simulink model "IEEE34bus_v2019b_Phasor_DPL"  (R2019b)
settings: Solver=VariableStepAuto  StartTime=0.0  StopTime=100  FixedStep=Ts  RelTol=1e-3
InitFcn:
  | a=1; % Loading Factor
  | Ts=0.1;% For Delay Blocks in Voltage Regulator Controls
  | 
  | % Simulation data for the IEEE 34 Node Test Feeder model
  | mi2km = 1.60934;%  miles to km conversion
  | ft2km = 0.0003048; % feet to km conversion
  | ms2F = 1*1e-6/(2*pi*60);% microsiemens to Farads conversion
  | 
  | %% Configuration 300 - series reactance - ohm/mile
  | R_300 = [1.3368 0.2101 0.2130;0.2101 1.3238 0.2066;0.2130 0.2066 1.3294];
  | X_300 = [1.3343 0.5779 0.5015;0.5779 1.3569 0.4591;0.5015 0.4591 1.3471];
  | % charging susceptance - microsiemens/mile
  | B_300 = [5.3350 -1.5313 -0.9943;-1.5313 5.0979 -0.6212;-0.9943 -0.6212 4.8880];
  | 
  | R_300 = R_300/mi2km;
  | L_300 = (X_300/(2*pi*60))/mi2km;
  | C_300 =(B_300*ms2F)/mi2km;
  | 
  | %% Configuration 301 - series reactance - ohm/mile
  | R_301 = [1.9300 0.2327 0.2359;0.2327 1.9157 0.2288;0.2359 0.2288 1.9219];
  | X_301 = [1.4115 0.6442 0.5691;0.6442 1.4281 0.5238;0.5691 0.5238 1.4209];
  | % charging susceptance - microsiemens/mile
  | B_301 = [5.1207 -1.4364 -0.9402;-1.4364 4.9055 -0.5951;-0.9402 -0.5951 4.7154];
  | 
  | R_301 = R_301/mi2km;
  | L_301 = (X_301/(2*pi*60))/mi2km;
  | C_301 =(B_301*ms2F)/mi2km;
  | 
  | 
  | %% Configuration 302 - series reactance - ohm/mile
  | R_302 = [2.7995 0 0;0 0 0;0 0 0];
  | X_302 = [1.4855 0 0;0 0 0;0 0 0];
  | % charging susceptance - microsiemens/mile
  | B_302 = [4.2251 0 0;0 0 0;0 0 0];
  | 
  | R_302 = R_302/mi2km;
  | L_302 = (X_302/(2*pi*60))/mi2km;
  | C_302 =(B_302*ms2F)/mi2km;
  | 
  | %% Configuration 303 - series reactance - ohm/mile
  | R_303 = [0 0 0;0 2.7995 0;0 0 0];
  | X_303 = [0 0 0;0 1.4855 0;0 0 0];
  | % charging susceptance - microsiemens/mile
  | B_303 = [0 0 0;0 4.2251 0;0 0 0];
  | 
  | R_303 = R_303/mi2km;
  | L_303 = (X_303/(2*pi*60))/mi2km;
  | C_303 =(B_303*ms2F)/mi2km;
  | 
  | %% Configuration 303 - series reactance - ohm/mile
  | R_304 = [0 0 0;0 1.9217 0;0 0 0];
  | X_304 = [0 0 0;0 1.4212 0;0 0 0];
  | % charging susceptance - microsiemens/mile
  | B_304 = [0 0 0;0 4.3637 0;0 0 0];
  | 
  | R_304 = R_304/mi2km;
  | L_304 = (X_304/(2*pi*60))/mi2km;
  | C_304 =(B_304*ms2F)/mi2km;
undefined symbols (not defined in the file or in its folder): find_system, j
libraries: powerlib x239, powerlib_meascontrol x22
(part 2 of 4)

== system IEEE34bus_v2019b_Phasor_DPL/810 ==
  1 : powerlib/Measurements/Three-Phase V-I Measurement  VoltageMeasurement=phase-to-ground  SetLabelV=on  LabelV=V810  Vpu=off  VpuLL=off  CurrentMeasurement=no  SetLabelI=on  LabelI=I634  Ipu=off  Pbase=100e6  Vbase=24900  OutputType=Complex  PhasorSimulation=on  PSBequivalent=0
      settings: SourceProductName=Simscape Electrical
  Ground{1..2,9,12} (4 alike) : powerlib/Elements/Ground  LConnTagsString=a
      settings: SourceProductName=Simscape Electrical
  b : PMIOPort  Side=Left
  B : PMIOPort  Port=2  Side=Right
  connections:
  Ground2/LConn1 -- 1/LConn3
  Ground1/LConn1 -- 1/RConn3
  b/RConn1 -- 1/RConn2
  1/RConn1 -- Ground9/LConn1
  Ground12/LConn1 -- 1/LConn1
  B/RConn1 -- 1/LConn2

== system IEEE34bus_v2019b_Phasor_DPL/818 ==
  1 : powerlib/Measurements/Three-Phase V-I Measurement  VoltageMeasurement=phase-to-ground  SetLabelV=on  LabelV=V818  Vpu=off  VpuLL=off  CurrentMeasurement=no  SetLabelI=on  LabelI=I634  Ipu=off  Pbase=100e6  Vbase=24900  OutputType=Complex  PhasorSimulation=on  PSBequivalent=0
      settings: SourceProductName=Simscape Electrical
  Ground{1..2,9,12} (4 alike) : powerlib/Elements/Ground  LConnTagsString=a
      settings: SourceProductName=Simscape Electrical
  a : PMIOPort  Side=Left
  A : PMIOPort  Port=2  Side=Right
  connections:
  Ground9/LConn1 -- 1/RConn2
  Ground12/LConn1 -- 1/LConn2
  Ground2/LConn1 -- 1/LConn3
  Ground1/LConn1 -- 1/RConn3
  A/RConn1 -- 1/LConn1
  a/RConn1 -- 1/RConn1

== system IEEE34bus_v2019b_Phasor_DPL/820 ==
  1 : powerlib/Measurements/Three-Phase V-I Measurement  VoltageMeasurement=phase-to-ground  SetLabelV=on  LabelV=V820  Vpu=off  VpuLL=off  CurrentMeasurement=no  SetLabelI=on  LabelI=I634  Ipu=off  Pbase=100e6  Vbase=24900  OutputType=Complex  PhasorSimulation=on  PSBequivalent=0
      settings: SourceProductName=Simscape Electrical
  Ground{1..2,9,12} (4 alike) : powerlib/Elements/Ground  LConnTagsString=a
      settings: SourceProductName=Simscape Electrical
  a : PMIOPort  Side=Left
  A : PMIOPort  Port=2  Side=Right
  connections:
  a/RConn1 -- 1/RConn1
  A/RConn1 -- 1/LConn1
  Ground1/LConn1 -- 1/RConn3
  Ground2/LConn1 -- 1/LConn3
  Ground12/LConn1 -- 1/LConn2
  Ground9/LConn1 -- 1/RConn2

== system IEEE34bus_v2019b_Phasor_DPL/822 ==
  1 : powerlib/Measurements/Three-Phase V-I Measurement  VoltageMeasurement=phase-to-ground  SetLabelV=on  LabelV=V822  Vpu=off  VpuLL=off  CurrentMeasurement=no  SetLabelI=on  LabelI=I634  Ipu=off  Pbase=100e6  Vbase=24900  OutputType=Complex  PhasorSimulation=on  PSBequivalent=0
      settings: SourceProductName=Simscape Electrical
  Ground{1..2,9,12} (4 alike) : powerlib/Elements/Ground  LConnTagsString=a
      settings: SourceProductName=Simscape Electrical
  a : PMIOPort  Side=Left
  A : PMIOPort  Port=2  Side=Right
  connections:
  Ground9/LConn1 -- 1/RConn2
  Ground12/LConn1 -- 1/LConn2
  Ground2/LConn1 -- 1/LConn3
  Ground1/LConn1 -- 1/RConn3
  A/RConn1 -- 1/LConn1
  a/RConn1 -- 1/RConn1

== system IEEE34bus_v2019b_Phasor_DPL/826 ==
  1 : powerlib/Measurements/Three-Phase V-I Measurement  VoltageMeasurement=phase-to-ground  SetLabelV=on  LabelV=V826  Vpu=off  VpuLL=off  CurrentMeasurement=no  SetLabelI=on  LabelI=I634  Ipu=off  Pbase=100e6  Vbase=24900  OutputType=Complex  PhasorSimulation=on  PSBequivalent=0
      settings: SourceProductName=Simscape Electrical
  Ground{1..2,9,12} (4 alike) : powerlib/Elements/Ground  LConnTagsString=a
      settings: SourceProductName=Simscape Electrical
  b : PMIOPort  Side=Left
  B : PMIOPort  Port=2  Side=Right
  connections:
  Ground1/LConn1 -- 1/RConn3
  Ground2/LConn1 -- 1/LConn3
  Ground9/LConn1 -- 1/RConn1
  b/RConn1 -- 1/RConn2
  Ground12/LConn1 -- 1/LConn1
  1/LConn2 -- B/RConn1

== system IEEE34bus_v2019b_Phasor_DPL/838 ==
  1 : powerlib/Measurements/Three-Phase V-I Measurement  VoltageMeasurement=phase-to-ground  SetLabelV=on  LabelV=V838  Vpu=off  VpuLL=off  CurrentMeasurement=no  SetLabelI=on  LabelI=I862  Ipu=off  Pbase=100e6  Vbase=24900  OutputType=Complex  PhasorSimulation=on  PSBequivalent=0
      settings: SourceProductName=Simscape Electrical
  Ground{1..2,9,12} (4 alike) : powerlib/Elements/Ground  LConnTagsString=a
      settings: SourceProductName=Simscape Electrical
  b : PMIOPort  Side=Left
  B : PMIOPort  Port=2  Side=Right
  connections:
  1/LConn2 -- B/RConn1
  Ground12/LConn1 -- 1/LConn1
  b/RConn1 -- 1/RConn2
  Ground9/LConn1 -- 1/RConn1
  Ground2/LConn1 -- 1/LConn3
  Ground1/LConn1 -- 1/RConn3

== system IEEE34bus_v2019b_Phasor_DPL/856 ==
  1 : powerlib/Measurements/Three-Phase V-I Measurement  VoltageMeasurement=phase-to-ground  SetLabelV=on  LabelV=V856  Vpu=off  VpuLL=off  CurrentMeasurement=no  SetLabelI=on  LabelI=I634  Ipu=off  Pbase=100e6  Vbase=24900  OutputType=Complex  PhasorSimulation=on  PSBequivalent=0
      settings: SourceProductName=Simscape Electrical
  Ground{1..2,9,12} (4 alike) : powerlib/Elements/Ground  LConnTagsString=a
      settings: SourceProductName=Simscape Electrical
  b : PMIOPort  Side=Left
  B : PMIOPort  Port=2  Side=Right
  connections:
  1/LConn2 -- B/RConn1
  Ground12/LConn1 -- 1/LConn1
  b/RConn1 -- 1/RConn2
  Ground9/LConn1 -- 1/RConn1
  Ground2/LConn1 -- 1/LConn3
  Ground1/LConn1 -- 1/RConn3

== system IEEE34bus_v2019b_Phasor_DPL/864 ==
  1 : powerlib/Measurements/Three-Phase V-I Measurement  VoltageMeasurement=phase-to-ground  SetLabelV=on  LabelV=V864  Vpu=off  VpuLL=off  CurrentMeasurement=no  SetLabelI=on  LabelI=I634  Ipu=off  Pbase=100e6  Vbase=24900  OutputType=Complex  PhasorSimulation=on  PSBequivalent=0
      settings: SourceProductName=Simscape Electrical
  Ground{1..2,9,12} (4 alike) : powerlib/Elements/Ground  LConnTagsString=a
      settings: SourceProductName=Simscape Electrical
  a : PMIOPort  Side=Left
  A : PMIOPort  Port=2  Side=Right
  connections:
  a/RConn1 -- 1/RConn1
  A/RConn1 -- 1/LConn1
  Ground1/LConn1 -- 1/RConn3
  Ground2/LConn1 -- 1/LConn3
  Ground12/LConn1 -- 1/LConn2
  Ground9/LConn1 -- 1/RConn2

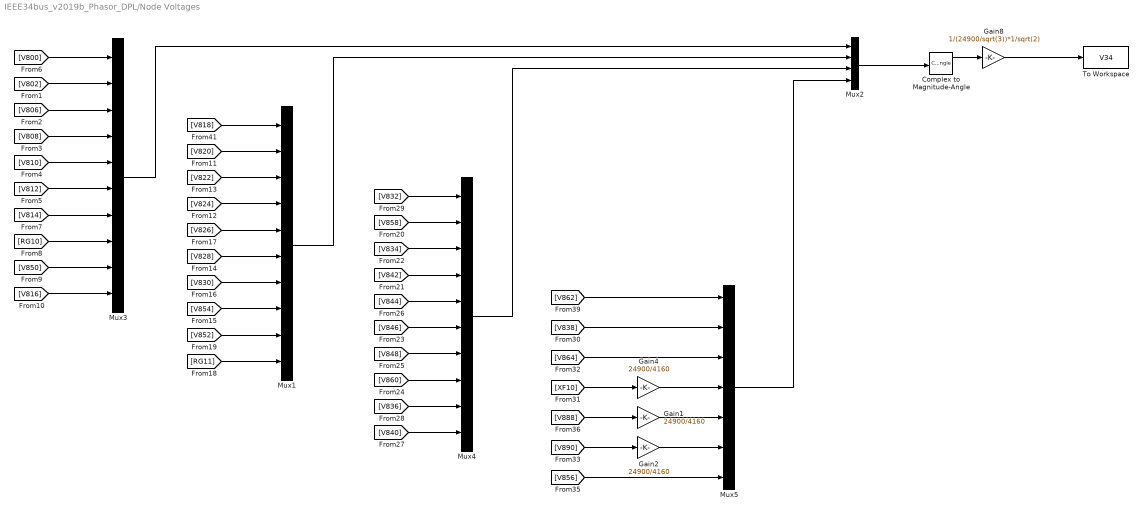
== system IEEE34bus_v2019b_Phasor_DPL/Node Voltages ==
  Complex to Magnitude-Angle : ComplexToMagnitudeAngle
  Gain1 : Gain  Gain=24900/4160
  Gain2 : Gain  Gain=24900/4160
  Gain4 : Gain  Gain=24900/4160
  Gain8 : Gain  Gain=1/(24900/sqrt(3))*1/sqrt(2)
  Mux1 : Mux  Inputs=10
  Mux2 : Mux
  Mux3 : Mux  Inputs=10
  Mux4 : Mux  Inputs=10
  Mux5 : Mux  Inputs=7
  To Workspace : ToWorkspace  VariableName=V34  SampleTime=0.1
  wires:
  [V800] -> Mux3/1
  [V802] -> Mux3/2
  [V806] -> Mux3/3
  [V808] -> Mux3/4
  [V810] -> Mux3/5
  [V812] -> Mux3/6
  [V814] -> Mux3/7
  [RG10] -> Mux3/8
  [V850] -> Mux3/9
  [V816] -> Mux3/10
  [V818] -> Mux1/1
  [V820] -> Mux1/2
  [V822] -> Mux1/3
  [V824] -> Mux1/4
  [V826] -> Mux1/5
  [V828] -> Mux1/6
  [V830] -> Mux1/7
  [V854] -> Mux1/8
  [V852] -> Mux1/9
  [RG11] -> Mux1/10
  [V832] -> Mux4/1
  [V858] -> Mux4/2
  [V834] -> Mux4/3
  [V842] -> Mux4/4
  [V844] -> Mux4/5
  [V846] -> Mux4/6
  [V848] -> Mux4/7
  [V860] -> Mux4/8
  [V836] -> Mux4/9
  [V840] -> Mux4/10
  [V862] -> Mux5/1
  [V838] -> Mux5/2
  [V864] -> Mux5/3
  [XF10] -> Gain4/1
  [V888] -> Gain1/1
  [V890] -> Gain2/1
  [V856] -> Mux5/7
  Mux3/1 -> Mux2/1
  Mux1/1 -> Mux2/2
  Mux4/1 -> Mux2/3
  Mux5/1 -> Mux2/4
  Gain4/1 -> Mux5/4
  Gain1/1 -> Mux5/5
  Gain2/1 -> Mux5/6
  Gain8/1 -> To Workspace/1
  Complex to Magnitude-Angle/1 -> Gain8/1
  Mux2/1 -> Complex to Magnitude-Angle/1

== system IEEE34bus_v2019b_Phasor_DPL/Regulator 1 ==
  Mux : Mux  Inputs=3
  Single Phase SVR_A : Subsystem  LoadFcn=find_system(gcs,'FollowLinks', 'on', 'LookUnderMasks', 'all');  mask(Single-Phase OLTC){pNom=5e6/3, fNom=60, vNom=24.9e3/sqrt(3), ctRatio=100, ptRatio=120, DeltaU=0.00625, TapMinMax=[-16 16], InitialTap=12, TapSelectionTime=8, RegulatorOn=on, Regulator=[122/120  2/120  2], Comp=[2.7 1.6]}
      mask prompts: pNom "Nominal Power (VA)"; fNom "Nominal Frequency (Hz)"; vNom "Nominal Voltage (Vrms)"; ctRatio "Primary CT Rating (A)"; ptRatio "PT Ratio"; DeltaU "Voltage Step Per Tap (pu)"; TapMinMax "Minimum and Maximum Tap Positions"; InitialTap "Initial Tap Position"; TapSelectionTime "Tap Selection Time (s)"; RegulatorOn "Voltage Regulator"; Regulator "Voltage Regulator [ Vref(pu) DeadBand(pu)  Delay(s)]"; Comp "Compensator Settings [R (V) X(V)]"
      mask help:
      | Models a single-phase On Load Tap Changer (OLTC). The single-phase primary of multi-tap winding is modeled with a Variable-Ratio Transformer block.
      |
      | The transformer voltage ratio U2/U1 (in pu) is given by:
      |                 U2/U1= 1/ (1+TapPosition*DeltaU)
      | Tap position 0 corresponds to nominal voltage ratio.
      |
      | When Voltage regulator is 'on',  voltage regulator asks for a tap change if:
      |                  abs(Vm-Vref)>DeadBand/2  during a time  t > Delay.
      |
      | where 'Vm' is voltage measured at regulating point and Vref is reference voltage.
      | With line drop compensation, Vm=Vsec-Isec(R+jX)
      mask init:
      | RegulatorVref=Regulator(1);
      | RegulatorDeadBand=Regulator(2);
      | RegulatorDelay=Regulator(3);
      | Rc=Comp(1);
      | Xc=Comp(2);
      mask TypeOptions RegulatorOn: off | on
      mask Callback RegulatorOn:
      | tempMaskVis=get_param(gcb,'MaskVisibilities');
      | if strcmp(get_param(gcb,'RegulatorOn'),'on')
      | 	tempMaskVis{11}='on';
      | 	set_param(gcb,'MaskVisibilities',tempMaskVis);
      | else
      | 	tempMaskVis{11}='off';
      | 	set_param(gcb,'MaskVisibilities',tempMaskVis);
      | end
      | if strcmp(get_param(gcb,'RegulatorOn'),'on')
      | 	tempMaskVis{12}='on';
      | 	set_param(gcb,'MaskVisibilities',tempMaskVis);
      | else
      | 	tempMaskVis{12}='off';
      | 	set_param(gcb,'MaskVisibilities',tempMaskVis);
      | end
      mask DialogControl Container8 Prompt: Setup
      mask DialogControl Container13 Prompt: Regulator Parameters
  Single Phase SVR_B : Subsystem  LoadFcn=find_system(gcs,'FollowLinks', 'on', 'LookUnderMasks', 'all');  mask(Single-Phase OLTC){pNom=5e6/3, fNom=60, vNom=24.9e3/sqrt(3), ctRatio=100, ptRatio=120, DeltaU=0.00625, TapMinMax=[-16 16], InitialTap=5, TapSelectionTime=8, RegulatorOn=on, Regulator=[122/120  2/120  2], Comp=[2.7 1.6]}
      mask prompts: pNom "Nominal Power (VA)"; fNom "Nominal Frequency (Hz)"; vNom "Nominal Voltage (Vrms)"; ctRatio "Primary CT Rating (A)"; ptRatio "PT Ratio"; DeltaU "Voltage Step Per Tap (pu)"; TapMinMax "Minimum and Maximum Tap Positions"; InitialTap "Initial Tap Position"; TapSelectionTime "Tap Selection Time (s)"; RegulatorOn "Voltage Regulator"; Regulator "Voltage Regulator [ Vref(pu) DeadBand(pu)  Delay(s)]"; Comp "Compensator Settings [R (V) X(V)]"
      mask help:
      | Models a single-phase On Load Tap Changer (OLTC). The single-phase primary of multi-tap winding is modeled with a Variable-Ratio Transformer block.
      |
      | The transformer voltage ratio U2/U1 (in pu) is given by:
      |                 U2/U1= 1/ (1+TapPosition*DeltaU)
      | Tap position 0 corresponds to nominal voltage ratio.
      |
      | When Voltage regulator is 'on',  voltage regulator asks for a tap change if:
      |                  abs(Vm-Vref)>DeadBand/2  during a time  t > Delay.
      |
      | where 'Vm' is voltage measured at regulating point and Vref is reference voltage.
      | With line drop compensation, Vm=Vsec-Isec(R+jX)
      mask init:
      | RegulatorVref=Regulator(1);
      | RegulatorDeadBand=Regulator(2);
      | RegulatorDelay=Regulator(3);
      | Rc=Comp(1);
      | Xc=Comp(2);
      mask TypeOptions RegulatorOn: off | on
      mask Callback RegulatorOn:
      | tempMaskVis=get_param(gcb,'MaskVisibilities');
      | if strcmp(get_param(gcb,'RegulatorOn'),'on')
      | 	tempMaskVis{11}='on';
      | 	set_param(gcb,'MaskVisibilities',tempMaskVis);
      | else
      | 	tempMaskVis{11}='off';
      | 	set_param(gcb,'MaskVisibilities',tempMaskVis);
      | end
      | if strcmp(get_param(gcb,'RegulatorOn'),'on')
      | 	tempMaskVis{12}='on';
      | 	set_param(gcb,'MaskVisibilities',tempMaskVis);
      | else
      | 	tempMaskVis{12}='off';
      | 	set_param(gcb,'MaskVisibilities',tempMaskVis);
      | end
      mask DialogControl Container8 Prompt: Setup
      mask DialogControl Container13 Prompt: Regulator Parameters
  Single Phase SVR_C : Subsystem  LoadFcn=find_system(gcs,'FollowLinks', 'on', 'LookUnderMasks', 'all');  mask(Single-Phase OLTC){pNom=5e6/3, fNom=60, vNom=24.9e3/sqrt(3), ctRatio=100, ptRatio=120, DeltaU=0.00625, TapMinMax=[-16 16], InitialTap=5, TapSelectionTime=8, RegulatorOn=on, Regulator=[122/120  2/120  2], Comp=[2.7 1.6]}
      mask prompts: pNom "Nominal Power (VA)"; fNom "Nominal Frequency (Hz)"; vNom "Nominal Voltage (Vrms)"; ctRatio "Primary CT Rating (A)"; ptRatio "PT Ratio"; DeltaU "Voltage Step Per Tap (pu)"; TapMinMax "Minimum and Maximum Tap Positions"; InitialTap "Initial Tap Position"; TapSelectionTime "Tap Selection Time (s)"; RegulatorOn "Voltage Regulator"; Regulator "Voltage Regulator [ Vref(pu) DeadBand(pu)  Delay(s)]"; Comp "Compensator Settings [R (V) X(V)]"
      mask help:
      | Models a single-phase On Load Tap Changer (OLTC). The single-phase primary of multi-tap winding is modeled with a Variable-Ratio Transformer block.
      |
      | The transformer voltage ratio U2/U1 (in pu) is given by:
      |                 U2/U1= 1/ (1+TapPosition*DeltaU)
      | Tap position 0 corresponds to nominal voltage ratio.
      |
      | When Voltage regulator is 'on',  voltage regulator asks for a tap change if:
      |                  abs(Vm-Vref)>DeadBand/2  during a time  t > Delay.
      |
      | where 'Vm' is voltage measured at regulating point and Vref is reference voltage.
      | With line drop compensation, Vm=Vsec-Isec(R+jX)
      mask init:
      | RegulatorVref=Regulator(1);
      | RegulatorDeadBand=Regulator(2);
      | RegulatorDelay=Regulator(3);
      | Rc=Comp(1);
      | Xc=Comp(2);
      mask TypeOptions RegulatorOn: off | on
      mask Callback RegulatorOn:
      | tempMaskVis=get_param(gcb,'MaskVisibilities');
      | if strcmp(get_param(gcb,'RegulatorOn'),'on')
      | 	tempMaskVis{11}='on';
      | 	set_param(gcb,'MaskVisibilities',tempMaskVis);
      | else
      | 	tempMaskVis{11}='off';
      | 	set_param(gcb,'MaskVisibilities',tempMaskVis);
      | end
      | if strcmp(get_param(gcb,'RegulatorOn'),'on')
      | 	tempMaskVis{12}='on';
      | 	set_param(gcb,'MaskVisibilities',tempMaskVis);
      | else
      | 	tempMaskVis{12}='off';
      | 	set_param(gcb,'MaskVisibilities',tempMaskVis);
      | end
      mask DialogControl Container8 Prompt: Setup
      mask DialogControl Container13 Prompt: Regulator Parameters
  A : PMIOPort  Side=Left
  a : PMIOPort  Port=2  Side=Right
  B : PMIOPort  Port=3  Side=Left
  b : PMIOPort  Port=4  Side=Right
  C : PMIOPort  Port=5  Side=Left
  c : PMIOPort  Port=6  Side=Right
  Tap : Outport
  wires:
  Mux/1 -> Tap/1
  Single Phase SVR_C/1(Tap) -> Mux/3
  Single Phase SVR_B/1(Tap) -> Mux/2
  Single Phase SVR_A/1(Tap) -> Mux/1
  connections:
  Single Phase SVR_C/RConn1 -- c/RConn1
  Single Phase SVR_C/LConn1 -- C/RConn1
  Single Phase SVR_B/RConn1 -- b/RConn1
  Single Phase SVR_B/LConn1 -- B/RConn1
  Single Phase SVR_A/LConn1 -- A/RConn1
  Single Phase SVR_A/RConn1 -- a/RConn1

== system IEEE34bus_v2019b_Phasor_DPL/Regulator 2 ==
  Mux : Mux  Inputs=3
  Single Phase SVR_A : Subsystem  LoadFcn=find_system(gcs,'FollowLinks', 'on', 'LookUnderMasks', 'all');  mask(Single-Phase OLTC){pNom=5e6/3, fNom=60, vNom=24.9e3/sqrt(3), ctRatio=100, ptRatio=120, DeltaU=0.00625, TapMinMax=[-16 16], InitialTap=13, TapSelectionTime=13, RegulatorOn=on, Regulator=[124/120  2/120  2], Comp=[2.5 1.5]}
      mask prompts: pNom "Nominal Power (VA)"; fNom "Nominal Frequency (Hz)"; vNom "Nominal Voltage (Vrms)"; ctRatio "Primary CT Rating (A)"; ptRatio "PT Ratio"; DeltaU "Voltage Step Per Tap (pu)"; TapMinMax "Minimum and Maximum Tap Positions"; InitialTap "Initial Tap Position"; TapSelectionTime "Tap Selection Time (s)"; RegulatorOn "Voltage Regulator"; Regulator "Voltage Regulator [ Vref(pu) DeadBand(pu)  Delay(s)]"; Comp "Compensator Settings [R (V) X(V)]"
      mask help:
      | Models a single-phase On Load Tap Changer (OLTC). The single-phase primary of multi-tap winding is modeled with a Variable-Ratio Transformer block.
      |
      | The transformer voltage ratio U2/U1 (in pu) is given by:
      |                 U2/U1= 1/ (1+TapPosition*DeltaU)
      | Tap position 0 corresponds to nominal voltage ratio.
      |
      | When Voltage regulator is 'on',  voltage regulator asks for a tap change if:
      |                  abs(Vm-Vref)>DeadBand/2  during a time  t > Delay.
      |
      | where 'Vm' is voltage measured at regulating point and Vref is reference voltage.
      | With line drop compensation, Vm=Vsec-Isec(R+jX)
      mask init:
      | RegulatorVref=Regulator(1);
      | RegulatorDeadBand=Regulator(2);
      | RegulatorDelay=Regulator(3);
      | Rc=Comp(1);
      | Xc=Comp(2);
      mask TypeOptions RegulatorOn: off | on
      mask Callback RegulatorOn:
      | tempMaskVis=get_param(gcb,'MaskVisibilities');
      | if strcmp(get_param(gcb,'RegulatorOn'),'on')
      | 	tempMaskVis{11}='on';
      | 	set_param(gcb,'MaskVisibilities',tempMaskVis);
      | else
      | 	tempMaskVis{11}='off';
      | 	set_param(gcb,'MaskVisibilities',tempMaskVis);
      | end
      | if strcmp(get_param(gcb,'RegulatorOn'),'on')
      | 	tempMaskVis{12}='on';
      | 	set_param(gcb,'MaskVisibilities',tempMaskVis);
      | else
      | 	tempMaskVis{12}='off';
      | 	set_param(gcb,'MaskVisibilities',tempMaskVis);
      | end
      mask DialogControl Container8 Prompt: Setup
      mask DialogControl Container13 Prompt: Regulator Parameters
  Single Phase SVR_B : Subsystem  LoadFcn=find_system(gcs,'FollowLinks', 'on', 'LookUnderMasks', 'all');  mask(Single-Phase OLTC){pNom=5e6/3, fNom=60, vNom=24.9e3/sqrt(3), ctRatio=100, ptRatio=120, DeltaU=0.00625, TapMinMax=[-16 16], InitialTap=11, TapSelectionTime=13, RegulatorOn=on, Regulator=[124/120  2/120  2], Comp=[2.5 1.5]}
      mask prompts: pNom "Nominal Power (VA)"; fNom "Nominal Frequency (Hz)"; vNom "Nominal Voltage (Vrms)"; ctRatio "Primary CT Rating (A)"; ptRatio "PT Ratio"; DeltaU "Voltage Step Per Tap (pu)"; TapMinMax "Minimum and Maximum Tap Positions"; InitialTap "Initial Tap Position"; TapSelectionTime "Tap Selection Time (s)"; RegulatorOn "Voltage Regulator"; Regulator "Voltage Regulator [ Vref(pu) DeadBand(pu)  Delay(s)]"; Comp "Compensator Settings [R (V) X(V)]"
      mask help:
      | Models a single-phase On Load Tap Changer (OLTC). The single-phase primary of multi-tap winding is modeled with a Variable-Ratio Transformer block.
      |
      | The transformer voltage ratio U2/U1 (in pu) is given by:
      |                 U2/U1= 1/ (1+TapPosition*DeltaU)
      | Tap position 0 corresponds to nominal voltage ratio.
      |
      | When Voltage regulator is 'on',  voltage regulator asks for a tap change if:
      |                  abs(Vm-Vref)>DeadBand/2  during a time  t > Delay.
      |
      | where 'Vm' is voltage measured at regulating point and Vref is reference voltage.
      | With line drop compensation, Vm=Vsec-Isec(R+jX)
      mask init:
      | RegulatorVref=Regulator(1);
      | RegulatorDeadBand=Regulator(2);
      | RegulatorDelay=Regulator(3);
      | Rc=Comp(1);
      | Xc=Comp(2);
      mask TypeOptions RegulatorOn: off | on
      mask Callback RegulatorOn:
      | tempMaskVis=get_param(gcb,'MaskVisibilities');
      | if strcmp(get_param(gcb,'RegulatorOn'),'on')
      | 	tempMaskVis{11}='on';
      | 	set_param(gcb,'MaskVisibilities',tempMaskVis);
      | else
      | 	tempMaskVis{11}='off';
      | 	set_param(gcb,'MaskVisibilities',tempMaskVis);
      | end
      | if strcmp(get_param(gcb,'RegulatorOn'),'on')
      | 	tempMaskVis{12}='on';
      | 	set_param(gcb,'MaskVisibilities',tempMaskVis);
      | else
      | 	tempMaskVis{12}='off';
      | 	set_param(gcb,'MaskVisibilities',tempMaskVis);
      | end
      mask DialogControl Container8 Prompt: Setup
      mask DialogControl Container13 Prompt: Regulator Parameters
  Single Phase SVR_C : Subsystem  LoadFcn=find_system(gcs,'FollowLinks', 'on', 'LookUnderMasks', 'all');  mask(Single-Phase OLTC){pNom=5e6/3, fNom=60, vNom=24.9e3/sqrt(3), ctRatio=100, ptRatio=120, DeltaU=0.00625, TapMinMax=[-16 16], InitialTap=12, TapSelectionTime=13, RegulatorOn=on, Regulator=[124/120  2/120  2], Comp=[2.5 1.5]}
      mask prompts: pNom "Nominal Power (VA)"; fNom "Nominal Frequency (Hz)"; vNom "Nominal Voltage (Vrms)"; ctRatio "Primary CT Rating (A)"; ptRatio "PT Ratio"; DeltaU "Voltage Step Per Tap (pu)"; TapMinMax "Minimum and Maximum Tap Positions"; InitialTap "Initial Tap Position"; TapSelectionTime "Tap Selection Time (s)"; RegulatorOn "Voltage Regulator"; Regulator "Voltage Regulator [ Vref(pu) DeadBand(pu)  Delay(s)]"; Comp "Compensator Settings [R (V) X(V)]"
      mask help:
      | Models a single-phase On Load Tap Changer (OLTC). The single-phase primary of multi-tap winding is modeled with a Variable-Ratio Transformer block.
      |
      | The transformer voltage ratio U2/U1 (in pu) is given by:
      |                 U2/U1= 1/ (1+TapPosition*DeltaU)
      | Tap position 0 corresponds to nominal voltage ratio.
      |
      | When Voltage regulator is 'on',  voltage regulator asks for a tap change if:
      |                  abs(Vm-Vref)>DeadBand/2  during a time  t > Delay.
      |
      | where 'Vm' is voltage measured at regulating point and Vref is reference voltage.
      | With line drop compensation, Vm=Vsec-Isec(R+jX)
      mask init:
      | RegulatorVref=Regulator(1);
      | RegulatorDeadBand=Regulator(2);
      | RegulatorDelay=Regulator(3);
      | Rc=Comp(1);
      | Xc=Comp(2);
      mask TypeOptions RegulatorOn: off | on
      mask Callback RegulatorOn:
      | tempMaskVis=get_param(gcb,'MaskVisibilities');
      | if strcmp(get_param(gcb,'RegulatorOn'),'on')
      | 	tempMaskVis{11}='on';
      | 	set_param(gcb,'MaskVisibilities',tempMaskVis);
      | else
      | 	tempMaskVis{11}='off';
      | 	set_param(gcb,'MaskVisibilities',tempMaskVis);
      | end
      | if strcmp(get_param(gcb,'RegulatorOn'),'on')
      | 	tempMaskVis{12}='on';
      | 	set_param(gcb,'MaskVisibilities',tempMaskVis);
      | else
      | 	tempMaskVis{12}='off';
      | 	set_param(gcb,'MaskVisibilities',tempMaskVis);
      | end
      mask DialogControl Container8 Prompt: Setup
      mask DialogControl Container13 Prompt: Regulator Parameters
  A : PMIOPort  Side=Left
  a : PMIOPort  Port=2  Side=Right
  B : PMIOPort  Port=3  Side=Left
  b : PMIOPort  Port=4  Side=Right
  C : PMIOPort  Port=5  Side=Left
  c : PMIOPort  Port=6  Side=Right
  Tap : Outport
  wires:
  Mux/1 -> Tap/1
  Single Phase SVR_C/1(Tap) -> Mux/3
  Single Phase SVR_B/1(Tap) -> Mux/2
  Single Phase SVR_A/1(Tap) -> Mux/1
  connections:
  Single Phase SVR_C/RConn1 -- c/RConn1
  Single Phase SVR_C/LConn1 -- C/RConn1
  Single Phase SVR_B/RConn1 -- b/RConn1
  Single Phase SVR_B/LConn1 -- B/RConn1
  Single Phase SVR_A/LConn1 -- A/RConn1
  Single Phase SVR_A/RConn1 -- a/RConn1

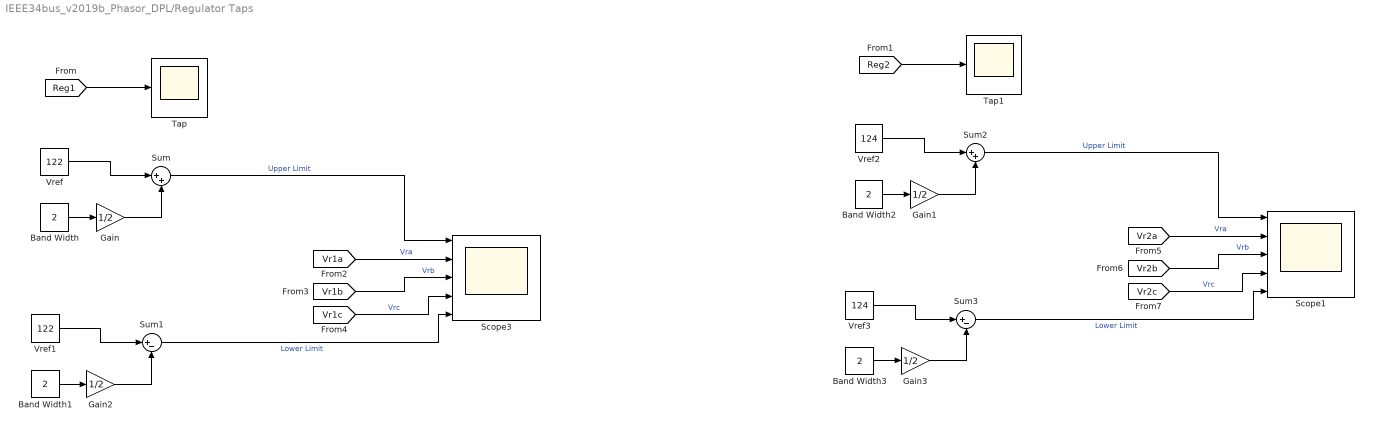
== system IEEE34bus_v2019b_Phasor_DPL/Regulator Taps ==
  Band Width{,1..3} (4 alike) : Constant  Value=2
  Gain{,1..3} (4 alike) : Gain  Gain=1/2
  Scope1 : Scope  NumInputPorts=5
  Scope3 : Scope  NumInputPorts=5
  Sum : Sum  Inputs=|++
  Sum1 : Sum  Inputs=|+-
  Sum2 : Sum  Inputs=|++
  Sum3 : Sum  Inputs=|+-
  Tap : Scope
  Tap1 : Scope
  Vref : Constant  Value=122
  Vref1 : Constant  Value=122
  Vref2 : Constant  Value=124
  Vref3 : Constant  Value=124
  wires:
  Vref/1 -> Sum/1
  Gain2/1 -> Sum1/2
  Band Width/1 -> Gain/1
  Gain/1 -> Sum/2
  [Reg1] -> Tap/1
  [Vr1c] -> Scope3/4  "Vrc"
  Band Width1/1 -> Gain2/1
  Sum/1 -> Scope3/1  "Upper Limit"
  Vref1/1 -> Sum1/1
  Sum1/1 -> Scope3/5  "Lower Limit"
  [Vr1b] -> Scope3/3  "Vrb"
  [Vr1a] -> Scope3/2  "Vra"
  [Vr2a] -> Scope1/2  "Vra"
  [Vr2b] -> Scope1/3  "Vrb"
  Sum3/1 -> Scope1/5  "Lower Limit"
  Vref3/1 -> Sum3/1
  Sum2/1 -> Scope1/1  "Upper Limit"
  Band Width3/1 -> Gain3/1
  [Vr2c] -> Scope1/4  "Vrc"
  [Reg2] -> Tap1/1
  Gain1/1 -> Sum2/2
  Band Width2/1 -> Gain1/1
  Gain3/1 -> Sum3/2
  Vref2/1 -> Sum2/1

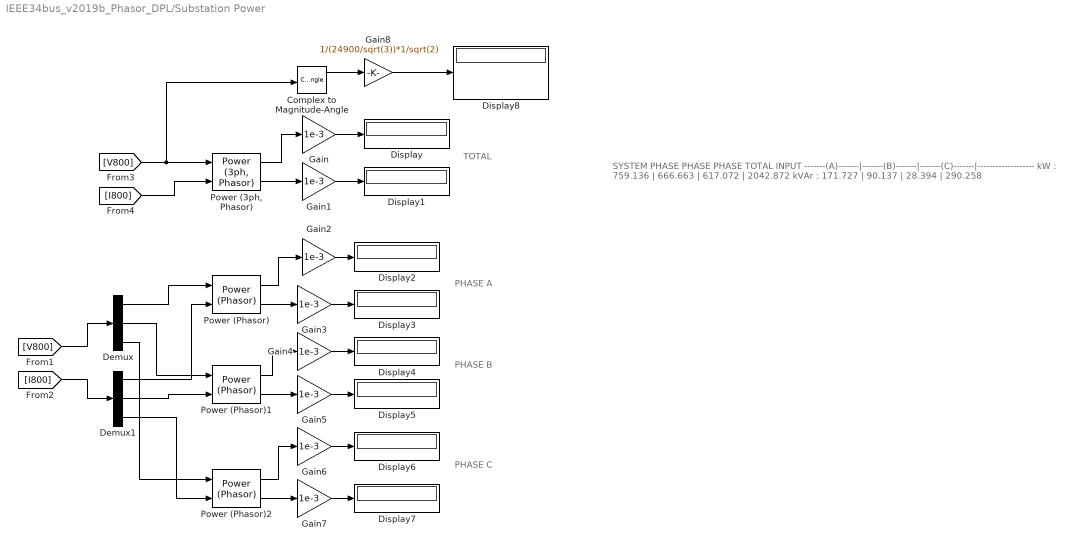
== system IEEE34bus_v2019b_Phasor_DPL/Substation Power ==
  note: SYSTEM PHASE PHASE PHASE TOTAL
      | INPUT -------(A)-------|-------(B)-------|-------(C)-------|-------------------
      | kW : 759.136 | 666.663 | 617.072 | 2042.872
      | kVAr : 171.727 | 90.137 | 28.394 | 290.258
  note: PHASE C
  note: PHASE A
  note: PHASE B
  note: TOTAL
  Complex to Magnitude-Angle : ComplexToMagnitudeAngle
  Demux : Demux  Outputs=3
  Demux1 : Demux  Outputs=3
  Display{,1..8} (9 alike) : Display
  Gain{,1..7} (8 alike) : Gain  Gain=1e-3
  Gain8 : Gain  Gain=1/(24900/sqrt(3))*1/sqrt(2)
  "Power (3ph, Phasor)" : powerlib_meascontrol/Measurements/Power (3ph, Phasor)
      settings: SourceProductName=Simscape Electrical  SourceProductBaseCode=PS
  Power (Phasor) : powerlib_meascontrol/Measurements/Power (Phasor)
      settings: SourceProductName=Simscape Electrical  SourceProductBaseCode=PS
  Power (Phasor)1 : powerlib_meascontrol/Measurements/Power (Phasor)
      settings: SourceProductName=Simscape Electrical  SourceProductBaseCode=PS
  Power (Phasor)2 : powerlib_meascontrol/Measurements/Power (Phasor)
      settings: SourceProductName=Simscape Electrical  SourceProductBaseCode=PS
  wires:
  [I800] -> "Power (3ph, Phasor)"/2
  "Power (3ph, Phasor)"/1 -> Gain/1
  "Power (3ph, Phasor)"/2 -> Gain1/1
  [V800] -> Demux/1
  [I800] -> Demux1/1
  Demux/1 -> Power (Phasor)/1
  Demux1/1 -> Power (Phasor)/2
  Demux/2 -> Power (Phasor)1/1
  Demux1/2 -> Power (Phasor)1/2
  Demux/3 -> Power (Phasor)2/1
  Demux1/3 -> Power (Phasor)2/2
  Power (Phasor)/1 -> Gain2/1
  Power (Phasor)/2 -> Gain3/1
  Power (Phasor)1/1 -> Gain4/1
  Power (Phasor)1/2 -> Gain5/1
  Power (Phasor)2/1 -> Gain6/1
  Power (Phasor)2/2 -> Gain7/1
  Gain/1 -> Display/1
  Gain1/1 -> Display1/1
  Gain2/1 -> Display2/1
  Gain3/1 -> Display3/1
  Gain4/1 -> Display4/1
  Gain5/1 -> Display5/1
  Gain6/1 -> Display6/1
  Gain7/1 -> Display7/1
  Complex to Magnitude-Angle/1 -> Gain8/1
  [V800] -> Complex to Magnitude-Angle/1, "Power (3ph, Phasor)"/1
  Gain8/1 -> Display8/1

== system IEEE34bus_v2019b_Phasor_DPL/Regulator 1/Single Phase SVR_A ==
  Line Drop Compensator : Subsystem
  Transformer with Taps : Subsystem
  Voltage Regulator Control : Subsystem
  S : PMIOPort  Tag=PMCPort  Side=Left
  L : PMIOPort  Tag=PMCPort  Port=2  Side=Right
  Tap : Outport  VectorParamsAs1DForOutWhenUnconnected=off
  tag scope: Vr1a=global
  wires:
  Line Drop Compensator/1(Vm) -> [Vr1a], Voltage Regulator Control/1(Vm)
  Voltage Regulator Control/1(Tap) -> Transformer with Taps/1(tap), Tap/1
  Transformer with Taps/1(Isec) -> Line Drop Compensator/1(Isec)
  Transformer with Taps/2(Vsec) -> Line Drop Compensator/2(Vsec)
  connections:
  Transformer with Taps/RConn1 -- L/RConn1
  Transformer with Taps/LConn1 -- S/RConn1

== system IEEE34bus_v2019b_Phasor_DPL/Regulator 1/Single Phase SVR_B ==
  Line Drop Compensator : Subsystem
  Transformer with Taps : Subsystem
  Voltage Regulator Control : Subsystem
  S : PMIOPort  Tag=PMCPort  Side=Left
  L : PMIOPort  Tag=PMCPort  Port=2  Side=Right
  Tap : Outport  VectorParamsAs1DForOutWhenUnconnected=off
  tag scope: Vr1b=global
  wires:
  Transformer with Taps/2(Vsec) -> Line Drop Compensator/2(Vsec)
  Transformer with Taps/1(Isec) -> Line Drop Compensator/1(Isec)
  Voltage Regulator Control/1(Tap) -> Transformer with Taps/1(tap), Tap/1
  Line Drop Compensator/1(Vm) -> [Vr1b], Voltage Regulator Control/1(Vm)
  connections:
  Transformer with Taps/LConn1 -- S/RConn1
  Transformer with Taps/RConn1 -- L/RConn1

== system IEEE34bus_v2019b_Phasor_DPL/Regulator 1/Single Phase SVR_C ==
  Line Drop Compensator : Subsystem
  Transformer with Taps : Subsystem
  Voltage Regulator Control : Subsystem
  S : PMIOPort  Tag=PMCPort  Side=Left
  L : PMIOPort  Tag=PMCPort  Port=2  Side=Right
  Tap : Outport  VectorParamsAs1DForOutWhenUnconnected=off
  tag scope: Vr1c=global
  wires:
  Line Drop Compensator/1(Vm) -> [Vr1c], Voltage Regulator Control/1(Vm)
  Voltage Regulator Control/1(Tap) -> Transformer with Taps/1(tap), Tap/1
  Transformer with Taps/1(Isec) -> Line Drop Compensator/1(Isec)
  Transformer with Taps/2(Vsec) -> Line Drop Compensator/2(Vsec)
  connections:
  Transformer with Taps/RConn1 -- L/RConn1
  Transformer with Taps/LConn1 -- S/RConn1

== system IEEE34bus_v2019b_Phasor_DPL/Regulator 2/Single Phase SVR_A ==
  Line Drop Compensator : Subsystem
  Transformer with Taps : Subsystem
  Voltage Regulator Control : Subsystem
  S : PMIOPort  Tag=PMCPort  Side=Left
  L : PMIOPort  Tag=PMCPort  Port=2  Side=Right
  Tap : Outport  VectorParamsAs1DForOutWhenUnconnected=off
  tag scope: Vr2a=global
  wires:
  Line Drop Compensator/1(Vm) -> [Vr2a], Voltage Regulator Control/1(Vm)
  Voltage Regulator Control/1(Tap) -> Transformer with Taps/1(tap), Tap/1
  Transformer with Taps/1(Isec) -> Line Drop Compensator/1(Isec)
  Transformer with Taps/2(Vsec) -> Line Drop Compensator/2(Vsec)
  connections:
  Transformer with Taps/RConn1 -- L/RConn1
  Transformer with Taps/LConn1 -- S/RConn1

== system IEEE34bus_v2019b_Phasor_DPL/Regulator 2/Single Phase SVR_B ==
  Line Drop Compensator : Subsystem
  Transformer with Taps : Subsystem
  Voltage Regulator Control : Subsystem
  S : PMIOPort  Tag=PMCPort  Side=Left
  L : PMIOPort  Tag=PMCPort  Port=2  Side=Right
  Tap : Outport  VectorParamsAs1DForOutWhenUnconnected=off
  tag scope: Vr2b=global
  wires:
  Transformer with Taps/2(Vsec) -> Line Drop Compensator/2(Vsec)
  Transformer with Taps/1(Isec) -> Line Drop Compensator/1(Isec)
  Voltage Regulator Control/1(Tap) -> Transformer with Taps/1(tap), Tap/1
  Line Drop Compensator/1(Vm) -> [Vr2b], Voltage Regulator Control/1(Vm)
  connections:
  Transformer with Taps/LConn1 -- S/RConn1
  Transformer with Taps/RConn1 -- L/RConn1

== system IEEE34bus_v2019b_Phasor_DPL/Regulator 2/Single Phase SVR_C ==
  Line Drop Compensator : Subsystem
  Transformer with Taps : Subsystem
  Voltage Regulator Control : Subsystem
  S : PMIOPort  Tag=PMCPort  Side=Left
  L : PMIOPort  Tag=PMCPort  Port=2  Side=Right
  Tap : Outport  VectorParamsAs1DForOutWhenUnconnected=off
  tag scope: Vr2c=global
  wires:
  Line Drop Compensator/1(Vm) -> [Vr2c], Voltage Regulator Control/1(Vm)
  Voltage Regulator Control/1(Tap) -> Transformer with Taps/1(tap), Tap/1
  Transformer with Taps/1(Isec) -> Line Drop Compensator/1(Isec)
  Transformer with Taps/2(Vsec) -> Line Drop Compensator/2(Vsec)
  connections:
  Transformer with Taps/RConn1 -- L/RConn1
  Transformer with Taps/LConn1 -- S/RConn1

== system IEEE34bus_v2019b_Phasor_DPL/Regulator 1/Single Phase SVR_A/Line Drop Compensator ==
  note: Vm=Vsec-Isec(Rc+jXc)
  Isec : Inport
  Vsec : Inport  Port=2
  Abs1 : Abs
  Gain4 : Gain  Gain=1/sqrt(2)
  Gain5 : Gain  Gain=Rc+j*Xc
  Gain6 : Gain  Gain=1/sqrt(2)
  Sum1 : Sum  Inputs=|+-
  Vm : Outport
  wires:
  Abs1/1 -> Vm/1
  Sum1/1 -> Abs1/1
  Isec/1 -> Gain4/1
  Vsec/1 -> Gain6/1
  Gain4/1 -> Gain5/1
  Gain6/1 -> Sum1/1
  Gain5/1 -> Sum1/2

== system IEEE34bus_v2019b_Phasor_DPL/Regulator 1/Single Phase SVR_A/Transformer with Taps ==
  note: Isec on CT Ratio base
  note: Vsec on Pt Ratio base
  tap : Inport
  "    " : Gain  Gain=(1/ptRatio)
  " 1" : Gain  Gain=(1/ctRatio)
  CT : powerlib/Measurements/Current Measurement  PhasorSimulation=on  OutputType=Complex  PSBequivalent=0
      settings: SourceProductName=Simscape Electrical
  Ground1 : powerlib/Elements/Ground  LConnTagsString=a
      settings: SourceProductName=Simscape Electrical
  Ground2 : powerlib/Elements/Ground  LConnTagsString=a
      settings: SourceProductName=Simscape Electrical
  Ground3 : powerlib/Elements/Ground  LConnTagsString=a
      settings: SourceProductName=Simscape Electrical
  Memory : Memory
  Memory1 : Memory
  PT : powerlib/Measurements/Voltage Measurement  PhasorSimulation=on  OutputType=Complex  PSBequivalent=0
      settings: SourceProductName=Simscape Electrical
  Tap Changing Transformer : Subsystem  mask(Tap Changing Transformer){}
      mask help: Implements a Tap changing two-winding ideal transformer with taps at secondary.
      mask Display:
      | A=[-85 -45 -44 -34 -26 -21 -20 -22 -28 -37 -47 -57 -63 -63 -54 -44 -34 -26 -21 -20 -22 -28 -37 -47 -57 -63 -63 -54 -44 -34 -26 -21 -20 -22 -28 -37 -47 -57 -63 -63 -54 -44 -34 -26 -21 -20 -22 -28 -37 -45 -45 -85];
      | B=[-50 -50 -50 -49 -45 -39 -33 -26 -21 -18 -17 -19 -22 -22 -26 -27 -25 -22 -16 -9 -3 2 6 6 4 1 1 -3 -4 -2 2 7 14 20 26 29 30 28 24 24 21 20 21 25 31 37 44 49 50 50 50 50];
      | C=[85 45 44 34 26 21 20 22 28 37 47 57 63 75 63 54 44 34 26 21 20 22 28 37 47 57 63 75 63 54 44 34 26 21 20 22 28 37 47 57 63 75 63 54 44 34 26 21 20 22 28 37 45 45 85];
      | D=[-50 -50 -50 -49 -45 -39 -33 -26 -21 -18 -17 -19 -22 -22 -22 -26 -27 -25 -22 -16 -9 -3 2 6 6 4 1 1 1 -3 -4 -2 2 7 14 20 26 29 30 28 24 24 24 21 20 21 25 31 37 44 49 50 50 50 50];
      | plot(-85,-100,85,100,A,B,C,D);
      | text(-50,-70, '1');text(40,-70, '2');
      | color('green')
      | port_label('Lconn',1,'+');port_label('Rconn',1,'+');
      | color('blue')
      | disp('N')
  L : PMIOPort  Tag=PMCPort  Side=Right
  S : PMIOPort  Port=2  Side=Left
  Isec : Outport
  Vsec : Outport  Port=2
  wires:
  tap/1 -> Tap Changing Transformer/1(Tap)
  Memory/1 -> Isec/1
  Memory1/1 -> Vsec/1
  " 1"/1 -> Memory/1
  CT/1 -> " 1"/1
  PT/1 -> "    "/1
  "    "/1 -> Memory1/1
  connections:
  Tap Changing Transformer/LConn2 -- Ground3/LConn1
  Tap Changing Transformer/LConn1 -- S/RConn1
  Tap Changing Transformer/RConn2 -- Ground2/LConn1
  CT/RConn1 -- L/RConn1
  PT/LConn1 -- CT/LConn1 -- Tap Changing Transformer/RConn1
  PT/LConn2 -- Ground1/LConn1

== system IEEE34bus_v2019b_Phasor_DPL/Regulator 1/Single Phase SVR_A/Voltage Regulator Control ==
  Vm : Inport
  Constant : Constant  Value=RegulatorOn
  Tap Changer Control : Subsystem  mask(Tap Changer Control){MinMaxTap=TapMinMax, InitialPosition=InitialTap, MecDelay=TapSelectionTime}
      mask prompts: MinMaxTap "Minimum and maximum tap number [ Min  Max ] :"; InitialPosition "Initial tap position"; MecDelay "Mechanical delay time"
      mask init:
      | if MecDelay<=0,
      | 	MecDelay=1/60;
      | end
  Voltage regulator : Subsystem  mask{Vref=RegulatorVref*120, DeadBand=RegulatorDeadBand*120, TimeDelay=RegulatorDelay}
      mask prompts: Vref "Vref (on 120v base)"; DeadBand "Deadband (on 120v base)"; TimeDelay "Time delay (s)"
  Tap : Outport
  wires:
  Voltage regulator/2(Down) -> Tap Changer Control/2("Down ")
  Tap Changer Control/1(TapNo) -> Tap/1  "Tap"
  Voltage regulator/1(Up) -> Tap Changer Control/1("Up ")
  Tap Changer Control/2(Ready) -> Voltage regulator/2(Ready)
  Constant/1 -> Voltage regulator/3(RegOn)
  Vm/1 -> Voltage regulator/1(Vmes (pu))

== system IEEE34bus_v2019b_Phasor_DPL/Regulator 1/Single Phase SVR_B/Line Drop Compensator ==
  note: Vm=Vsec-Isec(Rc+jXc)
  Isec : Inport
  Vsec : Inport  Port=2
  Abs1 : Abs
  Gain4 : Gain  Gain=1/sqrt(2)
  Gain5 : Gain  Gain=Rc+j*Xc
  Gain6 : Gain  Gain=1/sqrt(2)
  Sum1 : Sum  Inputs=|+-
  Vm : Outport
  wires:
  Abs1/1 -> Vm/1
  Sum1/1 -> Abs1/1
  Isec/1 -> Gain4/1
  Vsec/1 -> Gain6/1
  Gain4/1 -> Gain5/1
  Gain6/1 -> Sum1/1
  Gain5/1 -> Sum1/2

== system IEEE34bus_v2019b_Phasor_DPL/Regulator 1/Single Phase SVR_B/Transformer with Taps ==
  note: Isec on CT Ratio base
  note: Vsec on Pt Ratio base
  tap : Inport
  "    " : Gain  Gain=(1/ptRatio)
  " 1" : Gain  Gain=(1/ctRatio)
  CT : powerlib/Measurements/Current Measurement  PhasorSimulation=on  OutputType=Complex  PSBequivalent=0
      settings: SourceProductName=Simscape Electrical
  Ground1 : powerlib/Elements/Ground  LConnTagsString=a
      settings: SourceProductName=Simscape Electrical
  Ground2 : powerlib/Elements/Ground  LConnTagsString=a
      settings: SourceProductName=Simscape Electrical
  Ground3 : powerlib/Elements/Ground  LConnTagsString=a
      settings: SourceProductName=Simscape Electrical
  Memory : Memory
  Memory1 : Memory
  PT : powerlib/Measurements/Voltage Measurement  PhasorSimulation=on  OutputType=Complex  PSBequivalent=0
      settings: SourceProductName=Simscape Electrical
  Tap Changing Transformer : Subsystem  mask(Tap Changing Transformer){}
      mask help: Implements a Tap changing two-winding ideal transformer with taps at secondary.
      mask Display:
      | A=[-85 -45 -44 -34 -26 -21 -20 -22 -28 -37 -47 -57 -63 -63 -54 -44 -34 -26 -21 -20 -22 -28 -37 -47 -57 -63 -63 -54 -44 -34 -26 -21 -20 -22 -28 -37 -47 -57 -63 -63 -54 -44 -34 -26 -21 -20 -22 -28 -37 -45 -45 -85];
      | B=[-50 -50 -50 -49 -45 -39 -33 -26 -21 -18 -17 -19 -22 -22 -26 -27 -25 -22 -16 -9 -3 2 6 6 4 1 1 -3 -4 -2 2 7 14 20 26 29 30 28 24 24 21 20 21 25 31 37 44 49 50 50 50 50];
      | C=[85 45 44 34 26 21 20 22 28 37 47 57 63 75 63 54 44 34 26 21 20 22 28 37 47 57 63 75 63 54 44 34 26 21 20 22 28 37 47 57 63 75 63 54 44 34 26 21 20 22 28 37 45 45 85];
      | D=[-50 -50 -50 -49 -45 -39 -33 -26 -21 -18 -17 -19 -22 -22 -22 -26 -27 -25 -22 -16 -9 -3 2 6 6 4 1 1 1 -3 -4 -2 2 7 14 20 26 29 30 28 24 24 24 21 20 21 25 31 37 44 49 50 50 50 50];
      | plot(-85,-100,85,100,A,B,C,D);
      | text(-50,-70, '1');text(40,-70, '2');
      | color('green')
      | port_label('Lconn',1,'+');port_label('Rconn',1,'+');
      | color('blue')
      | disp('N')
  L : PMIOPort  Tag=PMCPort  Side=Right
  S : PMIOPort  Port=2  Side=Left
  Isec : Outport
  Vsec : Outport  Port=2
  wires:
  tap/1 -> Tap Changing Transformer/1(Tap)
  Memory/1 -> Isec/1
  Memory1/1 -> Vsec/1
  " 1"/1 -> Memory/1
  CT/1 -> " 1"/1
  PT/1 -> "    "/1
  "    "/1 -> Memory1/1
  connections:
  Tap Changing Transformer/LConn2 -- Ground3/LConn1
  Tap Changing Transformer/LConn1 -- S/RConn1
  Tap Changing Transformer/RConn2 -- Ground2/LConn1
  CT/RConn1 -- L/RConn1
  PT/LConn1 -- CT/LConn1 -- Tap Changing Transformer/RConn1
  PT/LConn2 -- Ground1/LConn1

== system IEEE34bus_v2019b_Phasor_DPL/Regulator 1/Single Phase SVR_B/Voltage Regulator Control ==
  Vm : Inport
  Constant : Constant  Value=RegulatorOn
  Tap Changer Control : Subsystem  mask(Tap Changer Control){MinMaxTap=TapMinMax, InitialPosition=InitialTap, MecDelay=TapSelectionTime}
      mask prompts: MinMaxTap "Minimum and maximum tap number [ Min  Max ] :"; InitialPosition "Initial tap position"; MecDelay "Mechanical delay time"
      mask init:
      | if MecDelay<=0,
      | 	MecDelay=1/60;
      | end
  Voltage regulator : Subsystem  mask{Vref=RegulatorVref*120, DeadBand=RegulatorDeadBand*120, TimeDelay=RegulatorDelay}
      mask prompts: Vref "Vref (on 120v base)"; DeadBand "Deadband (on 120v base)"; TimeDelay "Time delay (s)"
  Tap : Outport
  wires:
  Voltage regulator/2(Down) -> Tap Changer Control/2("Down ")
  Tap Changer Control/1(TapNo) -> Tap/1  "Tap"
  Voltage regulator/1(Up) -> Tap Changer Control/1("Up ")
  Tap Changer Control/2(Ready) -> Voltage regulator/2(Ready)
  Constant/1 -> Voltage regulator/3(RegOn)
  Vm/1 -> Voltage regulator/1(Vmes (pu))

== system IEEE34bus_v2019b_Phasor_DPL/Regulator 1/Single Phase SVR_C/Line Drop Compensator ==
  note: Vm=Vsec-Isec(Rc+jXc)
  Isec : Inport
  Vsec : Inport  Port=2
  Abs1 : Abs
  Gain4 : Gain  Gain=1/sqrt(2)
  Gain5 : Gain  Gain=Rc+j*Xc
  Gain6 : Gain  Gain=1/sqrt(2)
  Sum1 : Sum  Inputs=|+-
  Vm : Outport
  wires:
  Abs1/1 -> Vm/1
  Sum1/1 -> Abs1/1
  Isec/1 -> Gain4/1
  Vsec/1 -> Gain6/1
  Gain4/1 -> Gain5/1
  Gain6/1 -> Sum1/1
  Gain5/1 -> Sum1/2

== system IEEE34bus_v2019b_Phasor_DPL/Regulator 1/Single Phase SVR_C/Transformer with Taps ==
  note: Isec on CT Ratio base
  note: Vsec on Pt Ratio base
  tap : Inport
  "    " : Gain  Gain=(1/ptRatio)
  " 1" : Gain  Gain=(1/ctRatio)
  CT : powerlib/Measurements/Current Measurement  PhasorSimulation=on  OutputType=Complex  PSBequivalent=0
      settings: SourceProductName=Simscape Electrical
  Ground1 : powerlib/Elements/Ground  LConnTagsString=a
      settings: SourceProductName=Simscape Electrical
  Ground2 : powerlib/Elements/Ground  LConnTagsString=a
      settings: SourceProductName=Simscape Electrical
  Ground3 : powerlib/Elements/Ground  LConnTagsString=a
      settings: SourceProductName=Simscape Electrical
  Memory : Memory
  Memory1 : Memory
  PT : powerlib/Measurements/Voltage Measurement  PhasorSimulation=on  OutputType=Complex  PSBequivalent=0
      settings: SourceProductName=Simscape Electrical
  Tap Changing Transformer : Subsystem  mask(Tap Changing Transformer){}
      mask help: Implements a Tap changing two-winding ideal transformer with taps at secondary.
      mask Display:
      | A=[-85 -45 -44 -34 -26 -21 -20 -22 -28 -37 -47 -57 -63 -63 -54 -44 -34 -26 -21 -20 -22 -28 -37 -47 -57 -63 -63 -54 -44 -34 -26 -21 -20 -22 -28 -37 -47 -57 -63 -63 -54 -44 -34 -26 -21 -20 -22 -28 -37 -45 -45 -85];
      | B=[-50 -50 -50 -49 -45 -39 -33 -26 -21 -18 -17 -19 -22 -22 -26 -27 -25 -22 -16 -9 -3 2 6 6 4 1 1 -3 -4 -2 2 7 14 20 26 29 30 28 24 24 21 20 21 25 31 37 44 49 50 50 50 50];
      | C=[85 45 44 34 26 21 20 22 28 37 47 57 63 75 63 54 44 34 26 21 20 22 28 37 47 57 63 75 63 54 44 34 26 21 20 22 28 37 47 57 63 75 63 54 44 34 26 21 20 22 28 37 45 45 85];
      | D=[-50 -50 -50 -49 -45 -39 -33 -26 -21 -18 -17 -19 -22 -22 -22 -26 -27 -25 -22 -16 -9 -3 2 6 6 4 1 1 1 -3 -4 -2 2 7 14 20 26 29 30 28 24 24 24 21 20 21 25 31 37 44 49 50 50 50 50];
      | plot(-85,-100,85,100,A,B,C,D);
      | text(-50,-70, '1');text(40,-70, '2');
      | color('green')
      | port_label('Lconn',1,'+');port_label('Rconn',1,'+');
      | color('blue')
      | disp('N')
  L : PMIOPort  Tag=PMCPort  Side=Right
  S : PMIOPort  Port=2  Side=Left
  Isec : Outport
  Vsec : Outport  Port=2
  wires:
  tap/1 -> Tap Changing Transformer/1(Tap)
  Memory/1 -> Isec/1
  Memory1/1 -> Vsec/1
  " 1"/1 -> Memory/1
  CT/1 -> " 1"/1
  PT/1 -> "    "/1
  "    "/1 -> Memory1/1
  connections:
  Tap Changing Transformer/LConn2 -- Ground3/LConn1
  Tap Changing Transformer/LConn1 -- S/RConn1
  Tap Changing Transformer/RConn2 -- Ground2/LConn1
  CT/RConn1 -- L/RConn1
  PT/LConn1 -- CT/LConn1 -- Tap Changing Transformer/RConn1
  PT/LConn2 -- Ground1/LConn1

== system IEEE34bus_v2019b_Phasor_DPL/Regulator 1/Single Phase SVR_C/Voltage Regulator Control ==
  Vm : Inport
  Constant : Constant  Value=RegulatorOn
  Tap Changer Control : Subsystem  mask(Tap Changer Control){MinMaxTap=TapMinMax, InitialPosition=InitialTap, MecDelay=TapSelectionTime}
      mask prompts: MinMaxTap "Minimum and maximum tap number [ Min  Max ] :"; InitialPosition "Initial tap position"; MecDelay "Mechanical delay time"
      mask init:
      | if MecDelay<=0,
      | 	MecDelay=1/60;
      | end
  Voltage regulator : Subsystem  mask{Vref=RegulatorVref*120, DeadBand=RegulatorDeadBand*120, TimeDelay=RegulatorDelay}
      mask prompts: Vref "Vref (on 120v base)"; DeadBand "Deadband (on 120v base)"; TimeDelay "Time delay (s)"
  Tap : Outport
  wires:
  Voltage regulator/2(Down) -> Tap Changer Control/2("Down ")
  Tap Changer Control/1(TapNo) -> Tap/1  "Tap"
  Voltage regulator/1(Up) -> Tap Changer Control/1("Up ")
  Tap Changer Control/2(Ready) -> Voltage regulator/2(Ready)
  Constant/1 -> Voltage regulator/3(RegOn)
  Vm/1 -> Voltage regulator/1(Vmes (pu))

== system IEEE34bus_v2019b_Phasor_DPL/Regulator 2/Single Phase SVR_A/Line Drop Compensator ==
  note: Vm=Vsec-Isec(Rc+jXc)
  Isec : Inport
  Vsec : Inport  Port=2
  Abs1 : Abs
  Gain4 : Gain  Gain=1/sqrt(2)
  Gain5 : Gain  Gain=Rc+j*Xc
  Gain6 : Gain  Gain=1/sqrt(2)
  Sum1 : Sum  Inputs=|+-
  Vm : Outport
  wires:
  Abs1/1 -> Vm/1
  Sum1/1 -> Abs1/1
  Isec/1 -> Gain4/1
  Vsec/1 -> Gain6/1
  Gain4/1 -> Gain5/1
  Gain6/1 -> Sum1/1
  Gain5/1 -> Sum1/2

== system IEEE34bus_v2019b_Phasor_DPL/Regulator 2/Single Phase SVR_A/Transformer with Taps ==
  note: Isec on CT Ratio base
  note: Vsec on Pt Ratio base
  tap : Inport
  "    " : Gain  Gain=(1/ptRatio)
  " 1" : Gain  Gain=(1/ctRatio)
  CT : powerlib/Measurements/Current Measurement  PhasorSimulation=on  OutputType=Complex  PSBequivalent=0
      settings: SourceProductName=Simscape Electrical
  Ground1 : powerlib/Elements/Ground  LConnTagsString=a
      settings: SourceProductName=Simscape Electrical
  Ground2 : powerlib/Elements/Ground  LConnTagsString=a
      settings: SourceProductName=Simscape Electrical
  Ground3 : powerlib/Elements/Ground  LConnTagsString=a
      settings: SourceProductName=Simscape Electrical
  Memory : Memory
  Memory1 : Memory
  PT : powerlib/Measurements/Voltage Measurement  PhasorSimulation=on  OutputType=Complex  PSBequivalent=0
      settings: SourceProductName=Simscape Electrical
  Tap Changing Transformer : Subsystem  mask(Tap Changing Transformer){}
      mask help: Implements a Tap changing two-winding ideal transformer with taps at secondary.
      mask Display:
      | A=[-85 -45 -44 -34 -26 -21 -20 -22 -28 -37 -47 -57 -63 -63 -54 -44 -34 -26 -21 -20 -22 -28 -37 -47 -57 -63 -63 -54 -44 -34 -26 -21 -20 -22 -28 -37 -47 -57 -63 -63 -54 -44 -34 -26 -21 -20 -22 -28 -37 -45 -45 -85];
      | B=[-50 -50 -50 -49 -45 -39 -33 -26 -21 -18 -17 -19 -22 -22 -26 -27 -25 -22 -16 -9 -3 2 6 6 4 1 1 -3 -4 -2 2 7 14 20 26 29 30 28 24 24 21 20 21 25 31 37 44 49 50 50 50 50];
      | C=[85 45 44 34 26 21 20 22 28 37 47 57 63 75 63 54 44 34 26 21 20 22 28 37 47 57 63 75 63 54 44 34 26 21 20 22 28 37 47 57 63 75 63 54 44 34 26 21 20 22 28 37 45 45 85];
      | D=[-50 -50 -50 -49 -45 -39 -33 -26 -21 -18 -17 -19 -22 -22 -22 -26 -27 -25 -22 -16 -9 -3 2 6 6 4 1 1 1 -3 -4 -2 2 7 14 20 26 29 30 28 24 24 24 21 20 21 25 31 37 44 49 50 50 50 50];
      | plot(-85,-100,85,100,A,B,C,D);
      | text(-50,-70, '1');text(40,-70, '2');
      | color('green')
      | port_label('Lconn',1,'+');port_label('Rconn',1,'+');
      | color('blue')
      | disp('N')
  L : PMIOPort  Tag=PMCPort  Side=Right
  S : PMIOPort  Port=2  Side=Left
  Isec : Outport
  Vsec : Outport  Port=2
  wires:
  tap/1 -> Tap Changing Transformer/1(Tap)
  Memory/1 -> Isec/1
  Memory1/1 -> Vsec/1
  " 1"/1 -> Memory/1
  CT/1 -> " 1"/1
  PT/1 -> "    "/1
  "    "/1 -> Memory1/1
  connections:
  Tap Changing Transformer/LConn2 -- Ground3/LConn1
  Tap Changing Transformer/LConn1 -- S/RConn1
  Tap Changing Transformer/RConn2 -- Ground2/LConn1
  CT/RConn1 -- L/RConn1
  PT/LConn1 -- CT/LConn1 -- Tap Changing Transformer/RConn1
  PT/LConn2 -- Ground1/LConn1

== system IEEE34bus_v2019b_Phasor_DPL/Regulator 2/Single Phase SVR_A/Voltage Regulator Control ==
  Vm : Inport
  Constant : Constant  Value=RegulatorOn
  Tap Changer Control : Subsystem  mask(Tap Changer Control){MinMaxTap=TapMinMax, InitialPosition=InitialTap, MecDelay=TapSelectionTime}
      mask prompts: MinMaxTap "Minimum and maximum tap number [ Min  Max ] :"; InitialPosition "Initial tap position"; MecDelay "Mechanical delay time"
      mask init:
      | if MecDelay<=0,
      | 	MecDelay=1/60;
      | end
  Voltage regulator : Subsystem  mask{Vref=RegulatorVref*120, DeadBand=RegulatorDeadBand*120, TimeDelay=RegulatorDelay}
      mask prompts: Vref "Vref (on 120v base)"; DeadBand "Deadband (on 120v base)"; TimeDelay "Time delay (s)"
  Tap : Outport
  wires:
  Voltage regulator/2(Down) -> Tap Changer Control/2("Down ")
  Tap Changer Control/1(TapNo) -> Tap/1  "Tap"
  Voltage regulator/1(Up) -> Tap Changer Control/1("Up ")
  Tap Changer Control/2(Ready) -> Voltage regulator/2(Ready)
  Constant/1 -> Voltage regulator/3(RegOn)
  Vm/1 -> Voltage regulator/1(Vmes (pu))

== system IEEE34bus_v2019b_Phasor_DPL/Regulator 2/Single Phase SVR_B/Line Drop Compensator ==
  note: Vm=Vsec-Isec(Rc+jXc)
  Isec : Inport
  Vsec : Inport  Port=2
  Abs1 : Abs
  Gain4 : Gain  Gain=1/sqrt(2)
  Gain5 : Gain  Gain=Rc+j*Xc
  Gain6 : Gain  Gain=1/sqrt(2)
  Sum1 : Sum  Inputs=|+-
  Vm : Outport
  wires:
  Abs1/1 -> Vm/1
  Sum1/1 -> Abs1/1
  Isec/1 -> Gain4/1
  Vsec/1 -> Gain6/1
  Gain4/1 -> Gain5/1
  Gain6/1 -> Sum1/1
  Gain5/1 -> Sum1/2
